simulink model "cross_subsystem_line"  (Simulink 6.3)
settings: Solver=ode45  StartTime=0.0  StopTime=10.0  RelTol=1e-3
settings Model: LastModifiedBy=deissenb

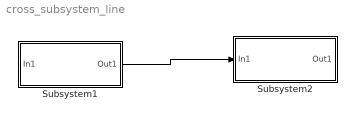
== system cross_subsystem_line ==
  Subsystem1 : Subsystem
  Subsystem2 : Subsystem
  wires:
  Subsystem1/1(Out1) -> Subsystem2/1(In1)

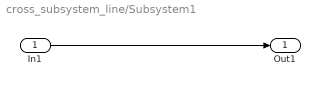
== system cross_subsystem_line/Subsystem1 ==
  In1 : Inport
  Out1 : Outport
  wires:
  In1/1 -> Out1/1

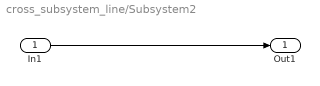
== system cross_subsystem_line/Subsystem2 ==
  In1 : Inport
  Out1 : Outport
  wires:
  In1/1 -> Out1/1
